simulink model "CascadeDCMotorController"  (Simulink 7.5)
settings: Solver=ode4  StartTime=0.0  StopTime=5  FixedStep=0.0001  RelTol=1e-3
values from neighbouring files (symbols this model uses):
  curKa = 1/curKi    (= 0.000176446721831)    [configure.m]
  curKff = 0.01    [configure.m]
  curKi = Wcc*motR    (= 5667.43314708)    [configure.m]
  curKp = Wcc*motL    (= 0.255097323471)    [configure.m]
  curMaxVolt = 50    [configure.m]
  motFm = 0.01    [configure.m]
  motJ = 4.27*0.001*0.01*0.01*10000    (= 0.00427)    [configure.m]
  motKb = 0    [configure.m]
  motKt = 24.4*0.001    (= 0.0244)    [configure.m]
  motL = 0.406*0.001    (= 0.000406)    [configure.m]
  motN = 1    [configure.m]
  motR = 9.02    [configure.m]
  posKa = 0    [configure.m]
  posKd = 1    [configure.m]
  posKi = 0    [configure.m]
  posKp = 30    [configure.m]
  posMaxVel = 100    [configure.m]
  velKa = 0.1    [configure.m]
  velKi = 0.1    [configure.m]
  velKp = 3    [configure.m]
  velKs = 0    [configure.m]
  velMaxCur = 10    [configure.m]
settings Model: Creator=HyungGi  LastModifiedBy=HyungGi

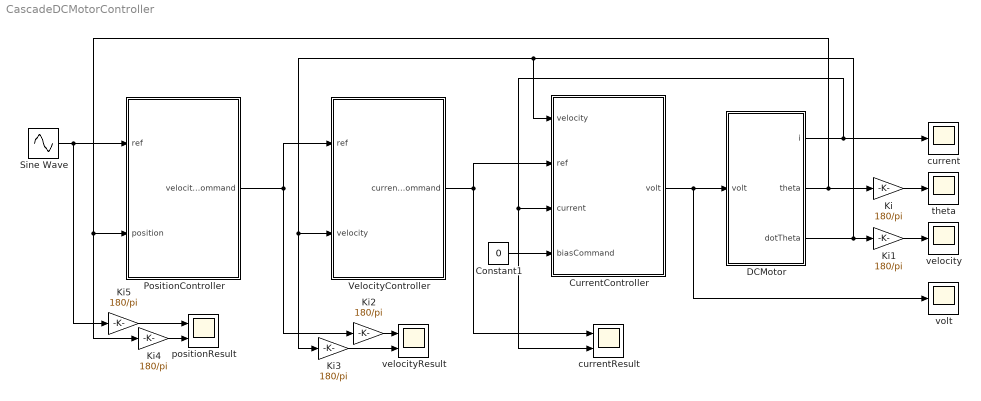
== system CascadeDCMotorController ==
  Constant1 : Constant  Value=0  OutDataType=fixdt(1, 16)  OutScaling=2^0
  CurrentController : Subsystem
  DCMotor : Subsystem
  Ki{,1..5} (6 alike) : Gain  Gain=180/pi  ParameterDataType=fixdt(1, 16)  ParameterScaling=2^0  OutDataType=fixdt(1, 16)  OutScaling=2^0
  PositionController : Subsystem
  Sine Wave : Sin  Amplitude=10*pi/180  Bias=0  Frequency=2*pi  Phase=0  Samples=10  SampleTime=0  Offset=0
  VelocityController : Subsystem
  current : Scope
      settings: YMin=-0.175  YMax=0.175
  currentResult : Scope  NumInputPorts=2
      settings: YMin=0~-5  YMax=11~5  SaveName=ScopeData3
  positionResult : Scope  NumInputPorts=2
      settings: YMin=-0.0365~-6.1e-005  YMax=-0.03375~-5.625e-005  SaveName=ScopeData6
  theta : Scope
      settings: YMin=0  YMax=11
  velocity : Scope
      settings: YMin=0  YMax=11  SaveName=ScopeData4
  velocityResult : Scope  NumInputPorts=2
      settings: YMin=-0.0365~-6.1e-005  YMax=-0.03375~-5.625e-005  SaveName=ScopeData5
  volt : Scope
      settings: YMin=0  YMax=11  SaveName=ScopeData2
  wires:
  CurrentController/1(volt) -> DCMotor/1(volt), volt/1
  DCMotor/1(i) -> current/1, CurrentController/3(current), currentResult/2
  DCMotor/3(dotTheta) -> CurrentController/1(velocity), VelocityController/2(velocity), Ki3/1, Ki1/1
  DCMotor/2(theta) -> Ki/1, PositionController/2(position), Ki4/1
  VelocityController/1(currentCommand) -> CurrentController/2(ref), currentResult/1
  Constant1/1 -> CurrentController/4(biasCommand)
  Ki/1 -> theta/1
  Ki1/1 -> velocity/1
  PositionController/1(velocityCommand) -> VelocityController/1(ref), Ki2/1
  Sine Wave/1 -> PositionController/1(ref), Ki5/1
  Ki2/1 -> velocityResult/1
  Ki3/1 -> velocityResult/2
  Ki4/1 -> positionResult/2
  Ki5/1 -> positionResult/1

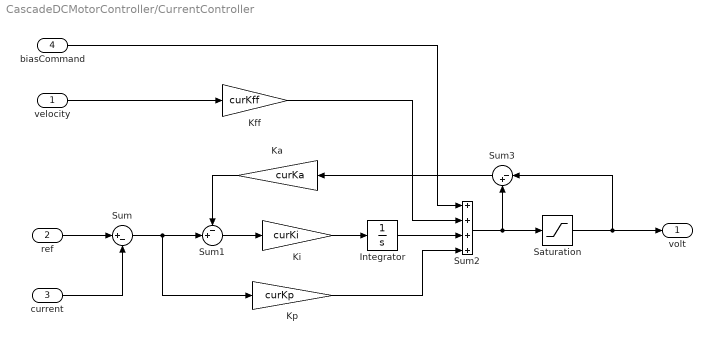
== system CascadeDCMotorController/CurrentController ==
  velocity : Inport  OutDataType=fixdt(1, 16)  OutScaling=2^0
  ref : Inport  Port=2  OutDataType=fixdt(1, 16)  OutScaling=2^0
  current : Inport  Port=3  OutDataType=fixdt(1, 16)  OutScaling=2^0
  biasCommand : Inport  Port=4  OutDataType=fixdt(1, 16)  OutScaling=2^0
  Integrator : Integrator
  Ka : Gain  Gain=curKa  ParameterDataType=fixdt(1, 16)  ParameterScaling=2^0  OutDataType=fixdt(1, 16)  OutScaling=2^0
  Kff : Gain  Gain=curKff  ParameterDataType=fixdt(1, 16)  ParameterScaling=2^0  OutDataType=fixdt(1, 16)  OutScaling=2^0
  Ki : Gain  Gain=curKi  ParameterDataType=fixdt(1, 16)  ParameterScaling=2^0  OutDataType=fixdt(1, 16)  OutScaling=2^0
  Kp : Gain  Gain=curKp  ParameterDataType=fixdt(1, 16)  ParameterScaling=2^0  OutDataType=fixdt(1, 16)  OutScaling=2^0
  Saturation : Saturate  UpperLimit=curMaxVolt  LowerLimit=-curMaxVolt  OutDataType=fixdt(1, 16)  OutScaling=2^0
  Sum : Sum  Inputs=|+-  OutDataType=fixdt(1, 16)  OutScaling=2^0
  Sum1 : Sum  Inputs=-+|  OutDataType=fixdt(1, 16)  OutScaling=2^0
  Sum2 : Sum  Inputs=++++  OutDataType=fixdt(1, 16)  OutScaling=2^0
  Sum3 : Sum  Inputs=|-+  OutDataType=fixdt(1, 16)  OutScaling=2^0
  volt : Outport  OutDataType=fixdt(1, 16)  OutScaling=2^0
  wires:
  ref/1 -> Sum/1
  current/1 -> Sum/2
  Sum/1 -> Sum1/2, Kp/1
  Sum1/1 -> Ki/1
  Ki/1 -> Integrator/1
  Kp/1 -> Sum2/4
  Integrator/1 -> Sum2/3
  velocity/1 -> Kff/1
  Ka/1 -> Sum1/1
  Kff/1 -> Sum2/2
  biasCommand/1 -> Sum2/1
  Sum2/1 -> Saturation/1, Sum3/2
  Saturation/1 -> volt/1, Sum3/1
  Sum3/1 -> Ka/1

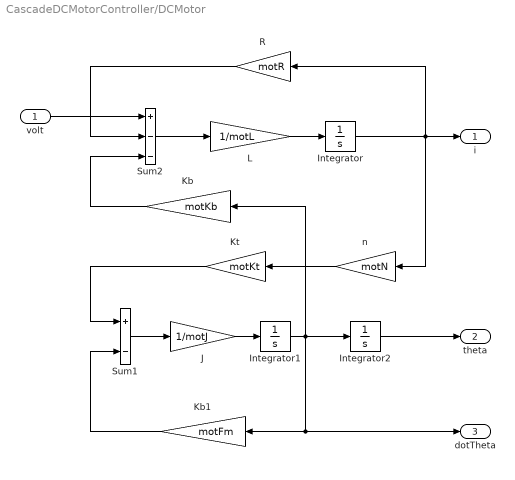
== system CascadeDCMotorController/DCMotor ==
  volt : Inport  OutDataType=fixdt(1, 16)  OutScaling=2^0
  Integrator : Integrator
  Integrator1 : Integrator
  Integrator2 : Integrator
  J : Gain  Gain=1/motJ  ParameterDataType=fixdt(1, 16)  ParameterScaling=2^0  OutDataType=fixdt(1, 16)  OutScaling=2^0
  Kb : Gain  Gain=motKb  ParameterDataType=fixdt(1, 16)  ParameterScaling=2^0  OutDataType=fixdt(1, 16)  OutScaling=2^0
  Kb1 : Gain  Gain=motFm  ParameterDataType=fixdt(1, 16)  ParameterScaling=2^0  OutDataType=fixdt(1, 16)  OutScaling=2^0
  Kt : Gain  Gain=motKt  ParameterDataType=fixdt(1, 16)  ParameterScaling=2^0  OutDataType=fixdt(1, 16)  OutScaling=2^0
  L : Gain  Gain=1/motL  ParameterDataType=fixdt(1, 16)  ParameterScaling=2^0  OutDataType=fixdt(1, 16)  OutScaling=2^0
  R : Gain  Gain=motR  ParameterDataType=fixdt(1, 16)  ParameterScaling=2^0  OutDataType=fixdt(1, 16)  OutScaling=2^0
  Sum1 : Sum  Inputs=+-  OutDataType=fixdt(1, 16)  OutScaling=2^0
  Sum2 : Sum  Inputs=+--  OutDataType=fixdt(1, 16)  OutScaling=2^0
  n : Gain  Gain=motN  ParameterDataType=fixdt(1, 16)  ParameterScaling=2^0  OutDataType=fixdt(1, 16)  OutScaling=2^0
  i : Outport  OutDataType=fixdt(1, 16)  OutScaling=2^0
  theta : Outport  Port=2  OutDataType=fixdt(1, 16)  OutScaling=2^0
  dotTheta : Outport  Port=3  OutDataType=fixdt(1, 16)  OutScaling=2^0
  wires:
  Integrator1/1 -> Integrator2/1, Kb/1, dotTheta/1, Kb1/1
  Integrator/1 -> i/1, R/1, n/1
  Integrator2/1 -> theta/1
  volt/1 -> Sum2/1
  R/1 -> Sum2/2
  Sum2/1 -> L/1
  Kb/1 -> Sum2/3
  L/1 -> Integrator/1
  Sum1/1 -> J/1
  n/1 -> Kt/1
  Kt/1 -> Sum1/1
  J/1 -> Integrator1/1
  Kb1/1 -> Sum1/2

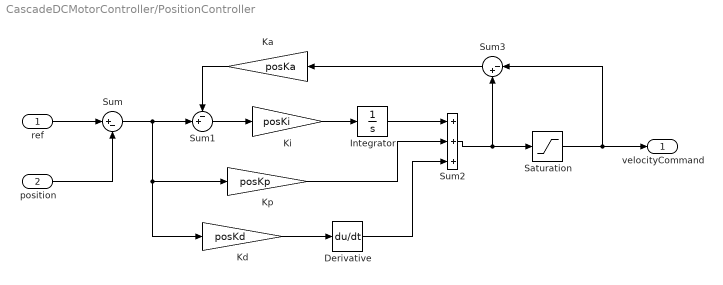
== system CascadeDCMotorController/PositionController ==
  ref : Inport  OutDataType=fixdt(1, 16)  OutScaling=2^0
  position : Inport  Port=2  OutDataType=fixdt(1, 16)  OutScaling=2^0
  Derivative : Derivative
  Integrator : Integrator
  Ka : Gain  Gain=posKa  ParameterDataType=fixdt(1, 16)  ParameterScaling=2^0  OutDataType=fixdt(1, 16)  OutScaling=2^0
  Kd : Gain  Gain=posKd  ParameterDataType=fixdt(1, 16)  ParameterScaling=2^0  OutDataType=fixdt(1, 16)  OutScaling=2^0
  Ki : Gain  Gain=posKi  ParameterDataType=fixdt(1, 16)  ParameterScaling=2^0  OutDataType=fixdt(1, 16)  OutScaling=2^0
  Kp : Gain  Gain=posKp  ParameterDataType=fixdt(1, 16)  ParameterScaling=2^0  OutDataType=fixdt(1, 16)  OutScaling=2^0
  Saturation : Saturate  UpperLimit=posMaxVel  LowerLimit=-posMaxVel  OutDataType=fixdt(1, 16)  OutScaling=2^0
  Sum : Sum  Inputs=|+-  OutDataType=fixdt(1, 16)  OutScaling=2^0
  Sum1 : Sum  Inputs=-+|  OutDataType=fixdt(1, 16)  OutScaling=2^0
  Sum2 : Sum  Inputs=+++  OutDataType=fixdt(1, 16)  OutScaling=2^0
  Sum3 : Sum  Inputs=|-+  OutDataType=fixdt(1, 16)  OutScaling=2^0
  velocityCommand : Outport  OutDataType=fixdt(1, 16)  OutScaling=2^0
  wires:
  Integrator/1 -> Sum2/1
  Sum3/1 -> Ka/1
  Saturation/1 -> Sum3/1, velocityCommand/1
  Sum2/1 -> Sum3/2, Saturation/1
  Ka/1 -> Sum1/1
  Kp/1 -> Sum2/2
  Ki/1 -> Integrator/1
  Sum1/1 -> Ki/1
  Sum/1 -> Sum1/2, Kp/1, Kd/1
  position/1 -> Sum/2
  ref/1 -> Sum/1
  Derivative/1 -> Sum2/3
  Kd/1 -> Derivative/1

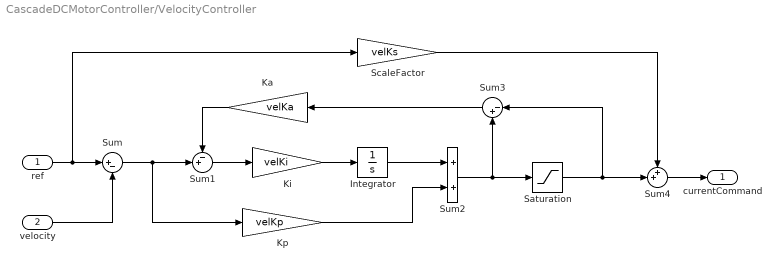
== system CascadeDCMotorController/VelocityController ==
  ref : Inport  OutDataType=fixdt(1, 16)  OutScaling=2^0
  velocity : Inport  Port=2  OutDataType=fixdt(1, 16)  OutScaling=2^0
  Integrator : Integrator
  Ka : Gain  Gain=velKa  ParameterDataType=fixdt(1, 16)  ParameterScaling=2^0  OutDataType=fixdt(1, 16)  OutScaling=2^0
  Ki : Gain  Gain=velKi  ParameterDataType=fixdt(1, 16)  ParameterScaling=2^0  OutDataType=fixdt(1, 16)  OutScaling=2^0
  Kp : Gain  Gain=velKp  ParameterDataType=fixdt(1, 16)  ParameterScaling=2^0  OutDataType=fixdt(1, 16)  OutScaling=2^0
  Saturation : Saturate  UpperLimit=velMaxCur  LowerLimit=-velMaxCur  OutDataType=fixdt(1, 16)  OutScaling=2^0
  ScaleFactor : Gain  Gain=velKs  ParameterDataType=fixdt(1, 16)  ParameterScaling=2^0  OutDataType=fixdt(1, 16)  OutScaling=2^0
  Sum : Sum  Inputs=|+-  OutDataType=fixdt(1, 16)  OutScaling=2^0
  Sum1 : Sum  Inputs=-+|  OutDataType=fixdt(1, 16)  OutScaling=2^0
  Sum2 : Sum  OutDataType=fixdt(1, 16)  OutScaling=2^0
  Sum3 : Sum  Inputs=|-+  OutDataType=fixdt(1, 16)  OutScaling=2^0
  Sum4 : Sum  Inputs=++|  OutDataType=fixdt(1, 16)  OutScaling=2^0
  currentCommand : Outport  OutDataType=fixdt(1, 16)  OutScaling=2^0
  wires:
  ref/1 -> Sum/1, ScaleFactor/1
  velocity/1 -> Sum/2
  Sum/1 -> Sum1/2, Kp/1
  Sum1/1 -> Ki/1
  Ki/1 -> Integrator/1
  Kp/1 -> Sum2/2
  Ka/1 -> Sum1/1
  Sum2/1 -> Saturation/1, Sum3/2
  Saturation/1 -> Sum3/1, Sum4/2
  Sum3/1 -> Ka/1
  Sum4/1 -> currentCommand/1
  ScaleFactor/1 -> Sum4/1
  Integrator/1 -> Sum2/1
